simulink model "HRD05"  (R2017b)
settings: Solver=ode8  StartTime=0.0  StopTime=Inf  FixedStep=0.001  RelTol=1e-3  EnableMultiTasking=on
undefined symbols (not defined in the file or in its folder): canChannel
libraries: c280xlib x7, canmsglib x4, canlib x3, c2806xlib x3, c2000lib x1, simulink x1, simulink_extras x1
settings Model: ExtModeTrigDuration=8  Creator=koffi  LastModifiedBy=Mark
settings OptimizationCC: LifeSpan=1  MaxStackSize=512
settings DebuggingCC: SFUnexpectedBacktrackingDiag=warning  SFNoUnconditionalDefaultTransitionDiag=warning  SFExecutionAtInitializationDiag=none
settings HardwareCC: ProdBitPerChar=16  ProdBitPerInt=16  ProdBitPerPointer=32  ProdBitPerSizeT=32  ProdBitPerPtrDiffT=32  ProdLargestAtomicInteger=Integer  ProdLargestAtomicFloat=None  ProdWordSize=16  ProdLongLongMode=on  ProdHWDeviceType=Texas Instruments->C2000
settings SFSimCC: MATLABDynamicMemAlloc=off
settings RTWCC: SystemTargetFile=ert.tlc  HardwareBoard=TI Piccolo F2806x (boot from flash)  TemplateMakefile=ert_default_tmf  GenerateReport=on  Toolchain=Texas Instruments Code Composer Studio (C2000)  IncludeHyperlinkInReport=on  LaunchReport=on  GenerateTraceInfo=on  GenerateTraceReport=on  GenerateTraceReportSl=on  GenerateTraceReportSf=on  GenerateTraceReportEml=on
settings CodeAppCC: ForceParamTrailComments=on  IgnoreCustomStorageClasses=off  OperatorAnnotations=on  SimulinkDataObjDesc=on  SFDataObjDesc=on  MATLABFcnDesc=on  InsertBlockDesc=on  StateflowObjectComments=on  MATLABSourceComments=on
settings ERTTargetCC: CodeReplacementLibrary=TI C28x  MultiwordLength=2048  ExtMode=on  ExtModeTransport=1  ExtModeMexFile=ext_serial_win32_comm  ExtModeMexArgs=1 7 114796
settings ConfigComp: CovMetricSettings=dw  CovHtmlReporting=on  CovSaveCumulativeToWorkspaceVar=on  CovSaveSingleToWorkspaceVar=on  CovExternalEMLEnable=off

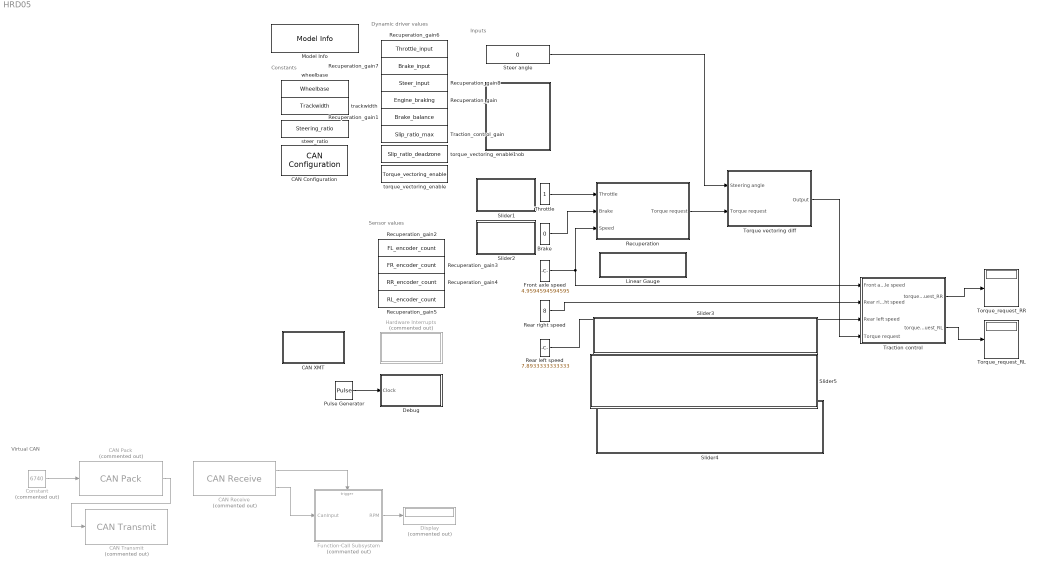
== system HRD05 ==
  note: Inputs
  note: Constants
  note: Dynamic driver values
  note: Sensor values
  note: Virtual CAN
  Brake : Constant  Value=0  OutDataTypeStr=double
  CAN Configuration : canlib/CAN Configuration  BlockHandle=5.0002  DeviceMenu=MathWorks Virtual 1 (Channel 1)  Device=MathWorks Virtual 1 (Channel 1)  ObjConstructor=canChannel('MathWorks','Virtual 1',1)  BusSpeed=500000  EnableBitParameters=off  AckMode=Normal
      settings: SourceProductName=Vehicle Network Toolbox  SourceProductBaseCode=VN
  CAN Pack : canmsglib/CAN Pack  Commented=on  CANdbFile=C:\HARD\HRD05-Control-system\config.dbc  MsgList=Engine_RPM  MsgName=Engine_RPM  MsgIDType=Standard (11-bit identifier)  MsgIdentifier=10  MsgLength=2  SignalInfo=Engine_RPM$0$15$1$2$1$0$1$0$0$32767$#  NSignals=1  StartBits=str2num('[int32(0)]')  SignalSizes=str2num('[int32(15)]')  ByteOrders=str2num('[int32(1)]')  DataTypes=str2num('[int32(2)]')  MultiplexTypes=str2num('[int32(1)]')  MultiplexValues=str2num('[double(0)]')  Factors=str2num('[double(1)]')  Offsets=str2num('[double(0)]')  Minimums=str2num('[double(0)]')  Maximums=str2num('[double(32767)]')  Remote=off  ApplyMinMax=off  BusOutput=off
      settings: SourceProductName=Simulink Real-Time  SourceProductBaseCode=XP  DataFormat=CANdb specified signals
  CAN Receive : canlib/CAN Receive  Commented=on  BlockHandle=7.0002  DeviceMenu=MathWorks Virtual 1 (Channel 1)  Device=MathWorks Virtual 1 (Channel 1)  ObjConstructor=canChannel('MathWorks','Virtual 1',1)  EnableStandardIDsFilter=off  StandardIDs=0  EnableExtendedIDsFilter=off  ExtendedIDs=0  SampleTime=0.01  MsgsPerTimestep=all  StdIDsCombo=Allow all  ExtIDsCombo=Allow all  InternalFilterUpdateStatus=on  BusOutput=off
      settings: SourceProductName=Vehicle Network Toolbox  SourceProductBaseCode=VN
  CAN Transmit : canlib/CAN Transmit  Commented=on  BlockHandle=8.0002  DeviceMenu=MathWorks Virtual 1 (Channel 1)  Device=MathWorks Virtual 1 (Channel 1)  ObjConstructor=canChannel('MathWorks','Virtual 1',1)  EnablePeriodicTransmit=off  MessagePeriod=1.000
      settings: SourceProductName=Vehicle Network Toolbox  SourceProductBaseCode=VN
  CAN XMT : Subsystem
  Constant : Constant  Commented=on  Value=6740
  Debug : Subsystem
  Display : Display  Commented=on
  Front axle speed : Constant  Value=4.9594594594595
  Function-Call Subsystem : Subsystem  Commented=on  TreatAsAtomicUnit=on
  Hardware Interrupts : Subsystem  Commented=on
  Knob : Subsystem  DialogController=hmiCreateDDGDialog  IsWebBlock=on  mask(MWDashboardBlock){webBlockId=45e470c3-09e4-44e8-ab03-ef5fc6b5f1f9, webBlockType=continuousknob, ShowInLibBrowser=on, ShowInitialText=on, HMISrcModelName=HRD05}
      mask prompts: webBlockId "WebBlock Id"; webBlockType "WebBlock Type"; HMISrcModelName "Source Model"
      mask help: SimulinkHMI:dialogs:ContinuousKnobDialogDesc
      mask Help: helpview([docroot '/mapfiles/simulink.map'], 'hmi_knob')
      mask Display:
      | if strcmp(get_param(bdroot(gcb),'BlockDiagramType'), 'library')
      |     image([(matlabroot) '/toolbox/simulink/hmi/icons/ContinuousKnob.png']);
      | end
  Linear Gauge : Subsystem  DialogController=hmiCreateDDGDialog  IsWebBlock=on  mask(MWDashboardBlock){webBlockId=bec7d255-bb7e-478d-9fdc-97f3e3b8b2d8, webBlockType=lineargauge, ShowInLibBrowser=on, ShowInitialText=on, HMISrcModelName=HRD05}
      mask prompts: webBlockId "WebBlock Id"; webBlockType "WebBlock Type"; HMISrcModelName "Source Model"
      mask help: SimulinkHMI:dialogs:LinearGaugeDialogDesc
      mask Help: helpview([docroot '/mapfiles/simulink.map'], 'hmi_linear_gauge')
      mask Display:
      | if strcmp(get_param(bdroot(gcb),'BlockDiagramType'), 'library')
      |     image([(matlabroot) '/toolbox/simulink/hmi/icons/LinearGauge.png']);
      | end
  Model Info : simulink/Model-Wide Utilities/Model Info  Frame=on  DisplayStringWithTags=|  HorizontalTextAlignment=Center  LeftAlignmentValue=0.5
      | Last edited by %<LastModifiedBy>,
      | %<LastModificationDate>
  Pulse Generator : DiscretePulseGenerator  PulseType=Time based  Period=1  PulseWidth=50
  Rear left speed : Constant  Value=7.8933333333333
  Rear right speed : Constant  Value=8
  Recuperation : Subsystem
  Recuperation_gain : DataStoreMemory  DataStoreName=Engine_braking  ReadBeforeWriteMsg=warning  WriteAfterWriteMsg=warning  WriteAfterReadMsg=warning  InitialValue=0.1  ShowAdditionalParam=off
  Recuperation_gain1 : DataStoreMemory  DataStoreName=Brake_balance  ReadBeforeWriteMsg=warning  WriteAfterWriteMsg=warning  WriteAfterReadMsg=warning  InitialValue=0.6  ShowAdditionalParam=off
  Recuperation_gain2 : DataStoreMemory  DataStoreName=FL_encoder_count  ReadBeforeWriteMsg=warning  WriteAfterWriteMsg=warning  WriteAfterReadMsg=warning  InitialValue=0.1  ShowAdditionalParam=off
  Recuperation_gain3 : DataStoreMemory  DataStoreName=FR_encoder_count  ReadBeforeWriteMsg=warning  WriteAfterWriteMsg=warning  WriteAfterReadMsg=warning  InitialValue=0.6  ShowAdditionalParam=off
  Recuperation_gain4 : DataStoreMemory  DataStoreName=RR_encoder_count  ReadBeforeWriteMsg=warning  WriteAfterWriteMsg=warning  WriteAfterReadMsg=warning  InitialValue=0.6  ShowAdditionalParam=off
  Recuperation_gain5 : DataStoreMemory  DataStoreName=RL_encoder_count  ReadBeforeWriteMsg=warning  WriteAfterWriteMsg=warning  WriteAfterReadMsg=warning  InitialValue=0.6  ShowAdditionalParam=off
  Recuperation_gain6 : DataStoreMemory  DataStoreName=Throttle_input  ReadBeforeWriteMsg=warning  WriteAfterWriteMsg=warning  WriteAfterReadMsg=warning  InitialValue=0.1  ShowAdditionalParam=off
  Recuperation_gain7 : DataStoreMemory  DataStoreName=Brake_input  ReadBeforeWriteMsg=warning  WriteAfterWriteMsg=warning  WriteAfterReadMsg=warning  InitialValue=0.1  ShowAdditionalParam=off
  Recuperation_gain8 : DataStoreMemory  DataStoreName=Steer_input  ReadBeforeWriteMsg=warning  WriteAfterWriteMsg=warning  WriteAfterReadMsg=warning  InitialValue=0.1  ShowAdditionalParam=off
  Slider1 : Subsystem  DialogController=hmiCreateDDGDialog  IsWebBlock=on  mask(MWDashboardBlock){webBlockId=6b16e8a2-996c-4c21-90ad-47c2870b8494, webBlockType=slider, ShowInLibBrowser=on, ShowInitialText=on, HMISrcModelName=HRD05}
      mask prompts: webBlockId "WebBlock Id"; webBlockType "WebBlock Type"; HMISrcModelName "Source Model"
      mask help: SimulinkHMI:dialogs:SliderDialogDesc
      mask Help: helpview([docroot '/mapfiles/simulink.map'], 'hmi_slider')
      mask Display:
      | if strcmp(get_param(bdroot(gcb),'BlockDiagramType'), 'library')
      |     image([(matlabroot) '/toolbox/simulink/hmi/icons/Slider.png']);
      | end
  Slider2 : Subsystem  DialogController=hmiCreateDDGDialog  IsWebBlock=on  mask(MWDashboardBlock){webBlockId=192e6944-36b0-45cd-ab7f-11e06ed1feff, webBlockType=slider, ShowInLibBrowser=on, ShowInitialText=on, HMISrcModelName=HRD05}
      mask prompts: webBlockId "WebBlock Id"; webBlockType "WebBlock Type"; HMISrcModelName "Source Model"
      mask help: SimulinkHMI:dialogs:SliderDialogDesc
      mask Help: helpview([docroot '/mapfiles/simulink.map'], 'hmi_slider')
      mask Display:
      | if strcmp(get_param(bdroot(gcb),'BlockDiagramType'), 'library')
      |     image([(matlabroot) '/toolbox/simulink/hmi/icons/Slider.png']);
      | end
  Slider3 : Subsystem  DialogController=hmiCreateDDGDialog  IsWebBlock=on  mask(MWDashboardBlock){webBlockId=7036d1ce-3a10-421e-b8b0-76df4fa24d80, webBlockType=slider, ShowInLibBrowser=on, ShowInitialText=on, HMISrcModelName=HRD05}
      mask prompts: webBlockId "WebBlock Id"; webBlockType "WebBlock Type"; HMISrcModelName "Source Model"
      mask help: SimulinkHMI:dialogs:SliderDialogDesc
      mask Help: helpview([docroot '/mapfiles/simulink.map'], 'hmi_slider')
      mask Display:
      | if strcmp(get_param(bdroot(gcb),'BlockDiagramType'), 'library')
      |     image([(matlabroot) '/toolbox/simulink/hmi/icons/Slider.png']);
      | end
  Slider4 : Subsystem  DialogController=hmiCreateDDGDialog  IsWebBlock=on  mask(MWDashboardBlock){webBlockId=54ff136d-0631-4094-b431-9d80d891858a, webBlockType=slider, ShowInLibBrowser=on, ShowInitialText=on, HMISrcModelName=HRD05}
      mask prompts: webBlockId "WebBlock Id"; webBlockType "WebBlock Type"; HMISrcModelName "Source Model"
      mask help: SimulinkHMI:dialogs:SliderDialogDesc
      mask Help: helpview([docroot '/mapfiles/simulink.map'], 'hmi_slider')
      mask Display:
      | if strcmp(get_param(bdroot(gcb),'BlockDiagramType'), 'library')
      |     image([(matlabroot) '/toolbox/simulink/hmi/icons/Slider.png']);
      | end
  Slider5 : Subsystem  DialogController=hmiCreateDDGDialog  IsWebBlock=on  mask(MWDashboardBlock){webBlockId=a28cbb47-1fb8-41d3-9559-6b9ff77cecec, webBlockType=slider, ShowInLibBrowser=on, ShowInitialText=on, HMISrcModelName=HRD05}
      mask prompts: webBlockId "WebBlock Id"; webBlockType "WebBlock Type"; HMISrcModelName "Source Model"
      mask help: SimulinkHMI:dialogs:SliderDialogDesc
      mask Help: helpview([docroot '/mapfiles/simulink.map'], 'hmi_slider')
      mask Display:
      | if strcmp(get_param(bdroot(gcb),'BlockDiagramType'), 'library')
      |     image([(matlabroot) '/toolbox/simulink/hmi/icons/Slider.png']);
      | end
  "Steer angle " : Constant  Value=0  OutDataTypeStr=double
  Throttle : Constant  OutDataTypeStr=double
  Torque vectoring diff : Subsystem  TreatAsAtomicUnit=on
  Torque_request_RL : Display
  Torque_request_RR : Display
  Traction control : Subsystem
  Traction_control_gain : DataStoreMemory  DataStoreName=Slip_ratio_max  ReadBeforeWriteMsg=warning  WriteAfterWriteMsg=warning  WriteAfterReadMsg=warning  InitialValue=2  ShowAdditionalParam=off
  steer_ratio : DataStoreMemory  DataStoreName=Steering_ratio  ReadBeforeWriteMsg=warning  WriteAfterWriteMsg=warning  WriteAfterReadMsg=warning  InitialValue=1.5  ShowAdditionalParam=off
  torque_vectoring_enable : DataStoreMemory  DataStoreName=Torque_vectoring_enable  ReadBeforeWriteMsg=warning  WriteAfterWriteMsg=warning  WriteAfterReadMsg=warning  InitialValue=1  ShowAdditionalParam=off
  torque_vectoring_enable1 : DataStoreMemory  DataStoreName=Slip_ratio_deadzone  ReadBeforeWriteMsg=warning  WriteAfterWriteMsg=warning  WriteAfterReadMsg=warning  InitialValue=1.12  ShowAdditionalParam=off
  trackwidth : DataStoreMemory  DataStoreName=Trackwidth  ReadBeforeWriteMsg=warning  WriteAfterWriteMsg=warning  WriteAfterReadMsg=warning  InitialValue=1.1  ShowAdditionalParam=off
  wheelbase : DataStoreMemory  DataStoreName=Wheelbase  ReadBeforeWriteMsg=warning  WriteAfterWriteMsg=warning  WriteAfterReadMsg=warning  InitialValue=1.5  ShowAdditionalParam=off
  wires:
  Brake/1 -> Recuperation/2(Brake)
  Throttle/1 -> Recuperation/1(Throttle)
  Torque vectoring diff/1("Output ") -> Traction control/4(Torque request)
  Front axle speed/1 -> Traction control/1(Front axle speed), Recuperation/3(Speed)
  Traction control/1("torque_request_RR ") -> Torque_request_RR/1
  Recuperation/1(Torque request) -> Torque vectoring diff/2(Torque request)
  Pulse Generator/1 -> Debug/1(Clock)
  CAN Receive/2 -> Function-Call Subsystem/1("CanInput ")
  Function-Call Subsystem/1(RPM) -> Display/1
  CAN Pack/1 -> CAN Transmit/1
  Constant/1 -> CAN Pack/1
  CAN Receive/1 -> Function-Call Subsystem/Trigger
  "Steer angle "/1 -> Torque vectoring diff/1(Steering angle)
  Rear left speed/1 -> Traction control/3(Rear left speed)
  Rear right speed/1 -> Traction control/2(Rear right speed)
  Traction control/2(torque_request_RL) -> Torque_request_RL/1

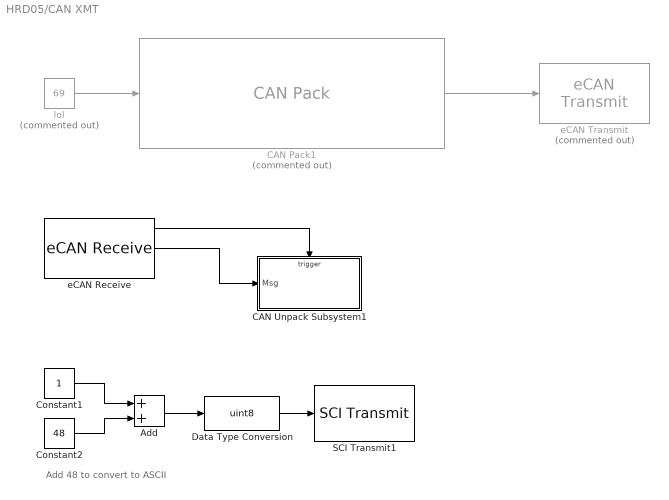
== system HRD05/CAN XMT ==
  note: Add 48 to convert to ASCII
  Add : Sum
  CAN Pack1 : canmsglib/CAN Pack  Commented=on  CANdbFile=C:\HARD\HRD05-Control-system\config.dbc  MsgList=Engine_RPM  MsgName=Engine_RPM  MsgIDType=Standard (11-bit identifier)  MsgIdentifier=10  MsgLength=2  SignalInfo=Engine_RPM$0$15$1$2$1$0$1$0$0$32767$#  NSignals=1  StartBits=str2num('[int32(0)]')  SignalSizes=str2num('[int32(15)]')  ByteOrders=str2num('[int32(1)]')  DataTypes=str2num('[int32(2)]')  MultiplexTypes=str2num('[int32(1)]')  MultiplexValues=str2num('[double(0)]')  Factors=str2num('[double(1)]')  Offsets=str2num('[double(0)]')  Minimums=str2num('[double(0)]')  Maximums=str2num('[double(32767)]')  Remote=off  ApplyMinMax=off  BusOutput=off
      settings: SourceProductName=Simulink Real-Time  DataFormat=raw data
  CAN Unpack Subsystem1 : Subsystem  TreatAsAtomicUnit=on
  Constant1 : Constant  SampleTime=-1
  Constant2 : Constant  Value=48
  Data Type Conversion : DataTypeConversion  OutDataTypeStr=uint8
  SCI Transmit1 : c280xlib/SCI Transmit  sciModule=A  dataHead='msg: '  dataTail=0  postInterrupt=off  numFifo=1
      settings: SourceProductName=Embedded Coder Support Package for Texas Instruments C2000 Processors
  eCAN Receive : c280xlib/eCAN Receive  chipFamily=C280x  useModule=eCAN_A  mailboxNo=0  messageID=18  messageType=Standard (11-bit identifier)  sampleTime=0.01  dataType=CAN_MESSAGE_TYPE  initValue=0  outputMessageLength=on  outputMessageTimeStamp=off  postInterrupt=off  interruptLine=0
      settings: SourceProductName=Embedded Coder Support Package for Texas Instruments C2000 Processors  SourceProductBaseCode=TIC2000
  eCAN Transmit : c280xlib/eCAN Transmit  Commented=on  chipFamily=C280x  useModule=eCAN_A  mailboxNo=1  messageID=bin2dec('111000111')  messageType=Standard (11-bit identifier)  enableBlockingMode=off  postInterrupt=off  interruptLine=0
      settings: SourceProductName=Embedded Coder Support Package for Texas Instruments C2000 Processors  SourceProductBaseCode=TIC2000
  "lol " : Constant  Commented=on  Value=69  OutDataTypeStr=uint16
  wires:
  "lol "/1 -> CAN Pack1/1
  CAN Pack1/1 -> eCAN Transmit/1
  eCAN Receive/2 -> CAN Unpack Subsystem1/1(Msg)
  eCAN Receive/1 -> CAN Unpack Subsystem1/Trigger
  Add/1 -> Data Type Conversion/1
  Data Type Conversion/1 -> SCI Transmit1/1
  Constant2/1 -> Add/2
  Constant1/1 -> Add/1

== system HRD05/Debug ==
  Clock : Inport
  Data Type Conversion : DataTypeConversion  OutDataTypeStr=uint8
  Digital Output : c2806xlib/Digital Output  GPIO_Number=GPIO32~GPIO39  GPIO_Bit0=off  GPIO_BIT0_Toggle=off  GPIO_Bit1=off  GPIO_BIT1_Toggle=off  GPIO_Bit2=on  GPIO_BIT2_Toggle=off  GPIO_Bit3=off  GPIO_BIT3_Toggle=off  GPIO_Bit4=off  GPIO_BIT4_Toggle=off  GPIO_Bit5=off  GPIO_BIT5_Toggle=off  GPIO_Bit6=off  GPIO_BIT6_Toggle=off  GPIO_Bit7=off  GPIO_BIT7_Toggle=off
      settings: SourceProductName=Embedded Coder Support Package for Texas Instruments C2000 Processors  SourceProductBaseCode=TIC2000
  wires:
  Clock/1 -> Data Type Conversion/1
  Data Type Conversion/1 -> Digital Output/1

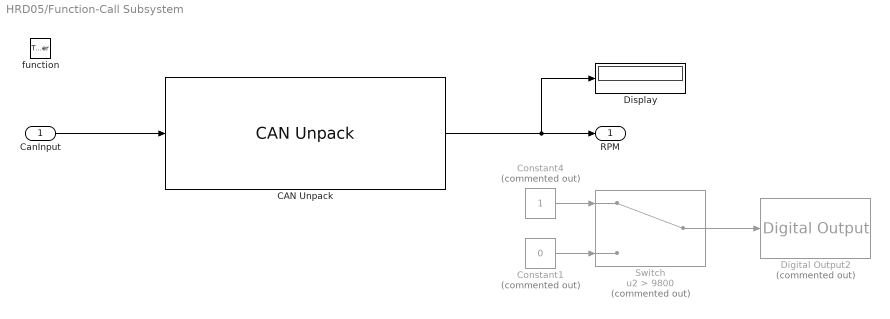
== system HRD05/Function-Call Subsystem ==
  "CanInput " : Inport
  function : TriggerPort  TriggerType=function-call  VariantControl=Variant
  CAN Unpack : canmsglib/CAN Unpack  CANdbFile=C:\HARD\HRD05-Control-system\config.dbc  MsgList=Engine_RPM  MsgName=Engine_RPM  MsgIDType=Standard (11-bit identifier)  MsgIdentifier=10  MsgLength=2  SignalInfo=Engine_RPM$0$15$1$2$1$0$1$0$0$32767$#  NSignals=1  IDPort=off  TimestampPort=off  ErrorPort=off  RemotePort=off  LengthPort=off  StatusPort=off  StartBits=str2num('[int32(0)]')  SignalSizes=str2num('[int32(15)]')  ByteOrders=str2num('[int32(1)]')  DataTypes=str2num('[int32(2)]')  MultiplexTypes=str2num('[int32(1)]')  MultiplexValues=str2num('[double(0)]')  Factors=str2num('[double(1)]')  Offsets=str2num('[double(0)]')  Minimums=str2num('[double(0)]')  Maximums=str2num('[double(32767)]')  ApplyMinMax=off
      settings: SourceProductName=Simulink Real-Time  SourceProductBaseCode=XP  DataFormat=CANdb specified signals
  Constant1 : Constant  Commented=on  Value=0  OutDataTypeStr=boolean
  Constant4 : Constant  Commented=on  OutDataTypeStr=boolean
  Digital Output2 : c2806xlib/Digital Output  Commented=on  GPIO_Number=GPIO32~GPIO39  GPIO_Bit0=off  GPIO_BIT0_Toggle=off  GPIO_Bit1=off  GPIO_BIT1_Toggle=off  GPIO_Bit2=on  GPIO_BIT2_Toggle=off  GPIO_Bit3=off  GPIO_BIT3_Toggle=off  GPIO_Bit4=off  GPIO_BIT4_Toggle=off  GPIO_Bit5=off  GPIO_BIT5_Toggle=off  GPIO_Bit6=off  GPIO_BIT6_Toggle=off  GPIO_Bit7=off  GPIO_BIT7_Toggle=off
      settings: SourceProductName=Embedded Coder Support Package for Texas Instruments C2000 Processors  SourceProductBaseCode=TIC2000
  Display : Display
  Switch : Switch  Commented=on  Criteria=u2 > Threshold  Threshold=9800
  RPM : Outport
  wires:
  "CanInput "/1 -> CAN Unpack/1
  CAN Unpack/1 -> Display/1, RPM/1
  Constant1/1 -> Switch/3
  Constant4/1 -> Switch/1
  Switch/1 -> Digital Output2/1

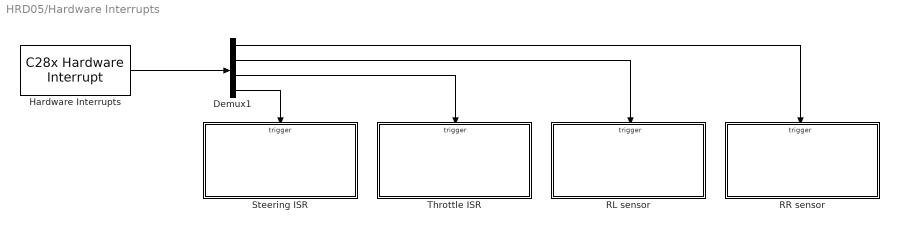
== system HRD05/Hardware Interrupts ==
  Demux1 : Demux
  Hardware Interrupts : c2000lib/Scheduling/C28x Hardware Interrupt  irqnumbers=[4 4 4 4]  pienumbers=[1 2 3 4]  irqpriorities=[25 25 2 2]  irqpreempts=[1 1 0 0]  showinput=off  dspchiptype=C280X
      settings: SourceProductName=Embedded Coder Support Package for Texas Instruments C2000 Processors  SourceProductBaseCode=TIC2000
  RL sensor : Subsystem  TreatAsAtomicUnit=on
  RR sensor : Subsystem  TreatAsAtomicUnit=on
  Steering ISR : Subsystem  TreatAsAtomicUnit=on
  Throttle ISR : Subsystem  TreatAsAtomicUnit=on
  wires:
  Hardware Interrupts/1 -> Demux1/1
  Demux1/1 -> RR sensor/Trigger
  Demux1/4 -> Steering ISR/Trigger
  Demux1/3 -> Throttle ISR/Trigger
  Demux1/2 -> RL sensor/Trigger

== system HRD05/Knob ==

== system HRD05/Linear Gauge ==

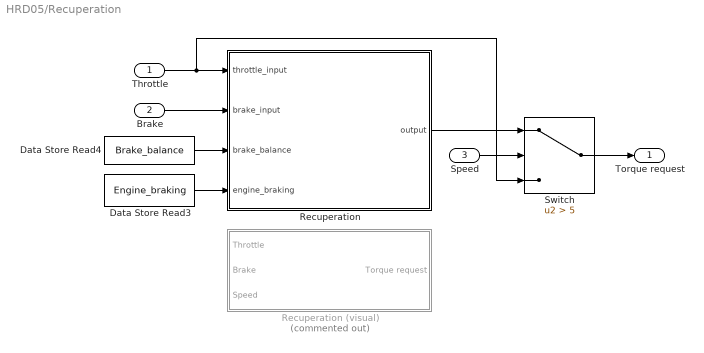
== system HRD05/Recuperation ==
  Throttle : Inport
  Brake : Inport  Port=2
  Speed : Inport  Port=3
  Data Store Read3 : DataStoreRead  DataStoreName=Engine_braking
  Data Store Read4 : DataStoreRead  DataStoreName=Brake_balance
  Recuperation : MATLAB Function  TreatAsAtomicUnit=on
  Recuperation (visual) : Subsystem  Commented=on
  Switch : Switch  Criteria=u2 > Threshold  Threshold=5
  Torque request : Outport
  wires:
  Throttle/1 -> Switch/3, Recuperation/1(throttle_input)
  Speed/1 -> Switch/2
  Recuperation/1(output) -> Switch/1
  Switch/1 -> Torque request/1
  Data Store Read4/1 -> Recuperation/3(brake_balance)
  Data Store Read3/1 -> Recuperation/4(engine_braking)
  Brake/1 -> Recuperation/2(brake_input)

== system HRD05/Slider1 ==

== system HRD05/Slider2 ==

== system HRD05/Slider3 ==

== system HRD05/Slider4 ==

== system HRD05/Slider5 ==

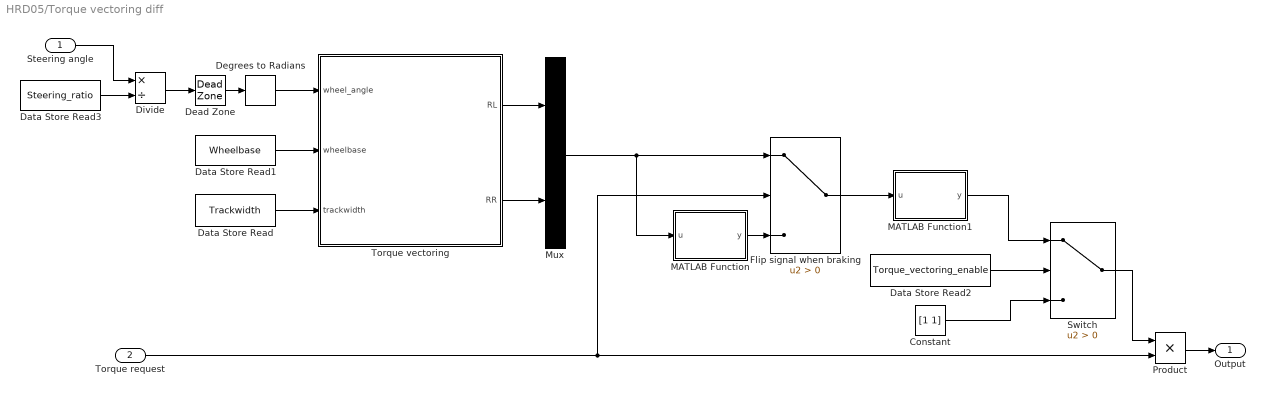
== system HRD05/Torque vectoring diff ==
  Steering angle : Inport
  Torque request : Inport  Port=2
  Constant : Constant  Value=[1 1]
  Data Store Read : DataStoreRead  DataStoreName=Trackwidth
  Data Store Read1 : DataStoreRead  DataStoreName=Wheelbase
  Data Store Read2 : DataStoreRead  DataStoreName=Torque_vectoring_enable
  Data Store Read3 : DataStoreRead  DataStoreName=Steering_ratio
  Dead Zone : DeadZone  LowerValue=-0.2  UpperValue=0.2  SaturateOnIntegerOverflow=on
  Degrees to Radians : simulink_extras/Transformations/Degrees to Radians
  Divide : Product  Inputs=*/
  Flip signal when braking : Switch  Criteria=u2 > Threshold
  MATLAB Function : MATLAB Function  TreatAsAtomicUnit=on
  MATLAB Function1 : MATLAB Function  TreatAsAtomicUnit=on
  Mux : Mux  Inputs=2
      settings: DisplayOption=signals
  Product : Product
  Switch : Switch  Criteria=u2 > Threshold
  Torque vectoring : MATLAB Function  TreatAsAtomicUnit=on
  "Output " : Outport  InitialOutput=[1 1]
  wires:
  Torque request/1 -> Flip signal when braking/2, Product/2
  MATLAB Function/1(y) -> Flip signal when braking/3
  Flip signal when braking/1 -> MATLAB Function1/1(u)
  Data Store Read2/1 -> Switch/2
  Constant/1 -> Switch/3
  Switch/1 -> Product/1
  MATLAB Function1/1(y) -> Switch/1
  Product/1 -> "Output "/1
  Data Store Read1/1 -> Torque vectoring/2(wheelbase)
  Dead Zone/1 -> Degrees to Radians/1
  Data Store Read/1 -> Torque vectoring/3(trackwidth)
  Torque vectoring/2(RR) -> Mux/2
  Torque vectoring/1(RL) -> Mux/1
  Degrees to Radians/1 -> Torque vectoring/1(wheel_angle)
  Mux/1 -> Flip signal when braking/1, MATLAB Function/1(u)
  Steering angle/1 -> Divide/1
  Data Store Read3/1 -> Divide/2
  Divide/1 -> Dead Zone/1

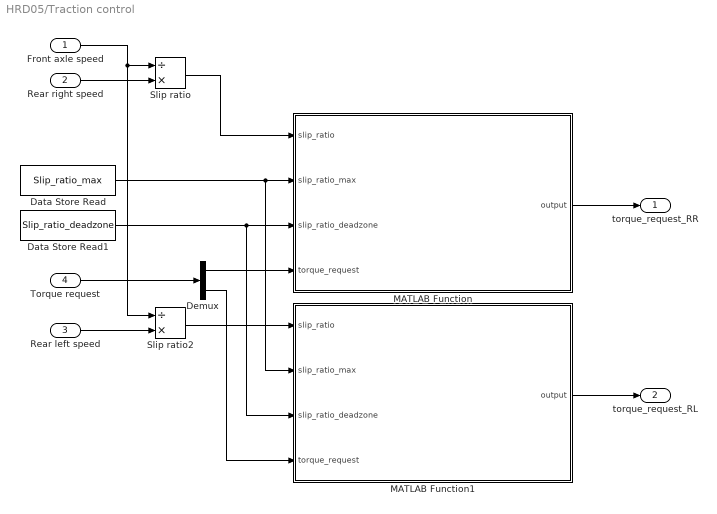
== system HRD05/Traction control ==
  Front axle speed : Inport
  Rear right speed : Inport  Port=2
  Rear left speed : Inport  Port=3
  Torque request : Inport  Port=4
  Data Store Read : DataStoreRead  DataStoreName=Slip_ratio_max
  Data Store Read1 : DataStoreRead  DataStoreName=Slip_ratio_deadzone
  Demux : Demux  Outputs=2
  MATLAB Function : MATLAB Function  TreatAsAtomicUnit=on
  MATLAB Function1 : MATLAB Function  TreatAsAtomicUnit=on
  Slip ratio : Product  Inputs=/*
  Slip ratio2 : Product  Inputs=/*
  "torque_request_RR " : Outport
  torque_request_RL : Outport  Port=2
  wires:
  MATLAB Function/1(output) -> "torque_request_RR "/1
  Torque request/1 -> Demux/1
  Front axle speed/1 -> Slip ratio2/1, Slip ratio/1
  Slip ratio/1 -> MATLAB Function/1(slip_ratio)
  Data Store Read/1 -> MATLAB Function1/2(slip_ratio_max), MATLAB Function/2(slip_ratio_max)
  Data Store Read1/1 -> MATLAB Function1/3(slip_ratio_deadzone), MATLAB Function/3(slip_ratio_deadzone)
  Demux/1 -> MATLAB Function/4(torque_request)
  Rear right speed/1 -> Slip ratio/2
  Slip ratio2/1 -> MATLAB Function1/1(slip_ratio)
  Rear left speed/1 -> Slip ratio2/2
  MATLAB Function1/1(output) -> torque_request_RL/1
  Demux/2 -> MATLAB Function1/4(torque_request)

== system HRD05/CAN XMT/CAN Unpack Subsystem1 ==
  Msg : Inport
  f : TriggerPort  TriggerType=function-call  VariantControl=Variant
  CAN Unpack : canmsglib/CAN Unpack  CANdbFile=C:\Users\josea\Desktop\C2000\CAN\Vector\RCDemo.dbc  MsgList=(none)  MsgName=Pedalbox  MsgIDType=Standard (11-bit identifier)  MsgIdentifier=18  MsgLength=2  SignalInfo=Throttle$0$8$2$1$1$0$1$0$0$255$#Brake$8$8$1$1$1$0$1$0$0$255$#  NSignals=2  IDPort=on  TimestampPort=on  ErrorPort=off  RemotePort=off  LengthPort=off  StatusPort=off  StartBits=str2num('[int32(0);int32(8)]')  SignalSizes=str2num('[int32(8);int32(8)]')  ByteOrders=str2num('[int32(2);int32(1)]')  DataTypes=str2num('[int32(1);int32(1)]')  MultiplexTypes=str2num('[int32(1);int32(1)]')  MultiplexValues=str2num('[double(0);double(0)]')  Factors=str2num('[double(1);double(1)]')  Offsets=str2num('[double(0);double(0)]')  Minimums=str2num('[double(0);double(0)]')  Maximums=str2num('[double(255);double(255)]')  ApplyMinMax=off
      settings: SourceProductName=Simulink Real-Time
  Digital Output : c2806xlib/Digital Output  Commented=on  GPIO_Number=GPIO32~GPIO39  GPIO_Bit0=off  GPIO_BIT0_Toggle=off  GPIO_Bit1=off  GPIO_BIT1_Toggle=off  GPIO_Bit2=on  GPIO_BIT2_Toggle=off  GPIO_Bit3=off  GPIO_BIT3_Toggle=off  GPIO_Bit4=off  GPIO_BIT4_Toggle=off  GPIO_Bit5=off  GPIO_BIT5_Toggle=off  GPIO_Bit6=off  GPIO_BIT6_Toggle=off  GPIO_Bit7=off  GPIO_BIT7_Toggle=off
      settings: SourceProductName=Embedded Coder Support Package for Texas Instruments C2000 Processors  SourceProductBaseCode=TIC2000
  wires:
  Msg/1 -> CAN Unpack/1
  CAN Unpack/1 -> Digital Output/1

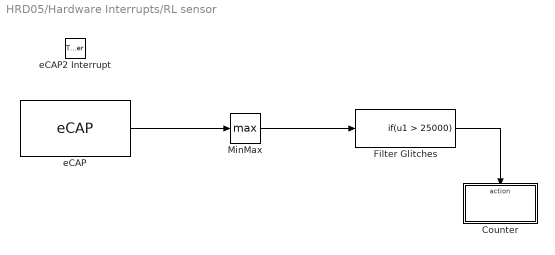
== system HRD05/Hardware Interrupts/RL sensor ==
  eCAP2 Interrupt : TriggerPort  TriggerType=function-call  VariantControl=Variant
  Counter : Subsystem  TreatAsAtomicUnit=on
  Filter Glitches : If  IfExpression=u1 > 25000  ShowElse=off
  MinMax : MinMax  Function=max
  eCAP : c280xlib/eCAP  operatingMode=eCAP  selectCAPx=eCAP2  offsetValue=0  counterSynIn=off  enableCounter=off  syncOutput=Disabled  sampleTime=-1  eventPrescaler=0  selectMode=Continuous  enableOneShot=off  stopValue=Capture Event 2  resetEv1Ts=off  ev1Polarity=Falling Edge  resetEv2Ts=on  ev2Polarity=Rising Edge  resetEv3Ts=off  ev3Polarity=Rising Edge  resetEv4Ts=on  ev4Polarity=Rising Edge  tSCntrDataType=uint32  capEvFlag=off  capFlagDataType=uint16  overFlowFlag=off  overFlowFlagDataType=uint16  periodUnit=Seconds  periodSource=Specify via dialog  waveformPeriod=0.001  dutyUnit=Percentages  dutySource=Specify via dialog  dutyCycle=50  outputPolarity=Active High  enableCEVT1Int=off  enableCEVT2Int=on  enableCEVT3Int=off  enableCEVT4Int=on  enableCTROVFInt=off  enablePRDInt=off  enableCMPInt=off
      settings: SourceProductName=Embedded Coder Support Package for Texas Instruments C2000 Processors  SourceProductBaseCode=TIC2000
  wires:
  eCAP/1 -> MinMax/1
  MinMax/1 -> Filter Glitches/1
  Filter Glitches/1 -> Counter/Action

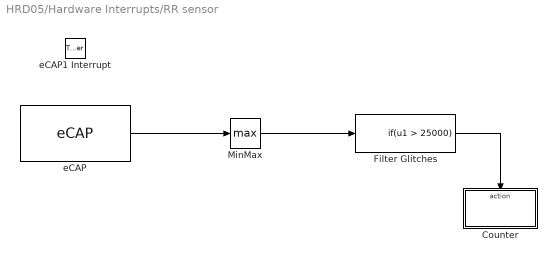
== system HRD05/Hardware Interrupts/RR sensor ==
  eCAP1 Interrupt : TriggerPort  TriggerType=function-call  VariantControl=Variant
  Counter : Subsystem  TreatAsAtomicUnit=on
  Filter Glitches : If  IfExpression=u1 > 25000  ShowElse=off
  MinMax : MinMax  Function=max
  eCAP : c280xlib/eCAP  operatingMode=eCAP  selectCAPx=eCAP1  offsetValue=0  counterSynIn=off  enableCounter=off  syncOutput=Disabled  sampleTime=-1  eventPrescaler=0  selectMode=Continuous  enableOneShot=off  stopValue=Capture Event 2  resetEv1Ts=off  ev1Polarity=Falling Edge  resetEv2Ts=on  ev2Polarity=Rising Edge  resetEv3Ts=off  ev3Polarity=Rising Edge  resetEv4Ts=on  ev4Polarity=Rising Edge  tSCntrDataType=uint32  capEvFlag=off  capFlagDataType=uint16  overFlowFlag=off  overFlowFlagDataType=uint16  periodUnit=Seconds  periodSource=Specify via dialog  waveformPeriod=0.001  dutyUnit=Percentages  dutySource=Specify via dialog  dutyCycle=50  outputPolarity=Active High  enableCEVT1Int=off  enableCEVT2Int=on  enableCEVT3Int=off  enableCEVT4Int=on  enableCTROVFInt=off  enablePRDInt=off  enableCMPInt=off
      settings: SourceProductName=Embedded Coder Support Package for Texas Instruments C2000 Processors  SourceProductBaseCode=TIC2000
  wires:
  Filter Glitches/1 -> Counter/Action
  MinMax/1 -> Filter Glitches/1
  eCAP/1 -> MinMax/1

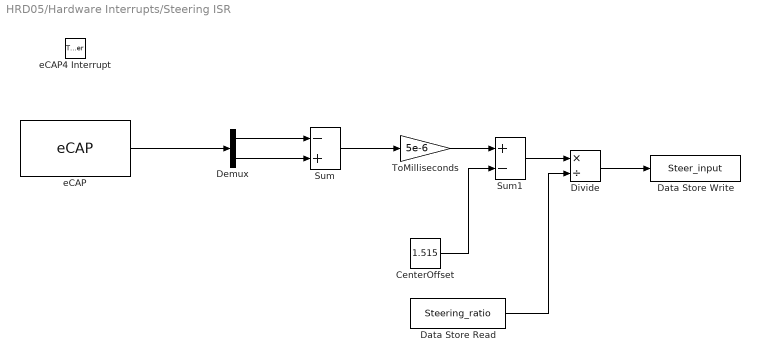
== system HRD05/Hardware Interrupts/Steering ISR ==
  eCAP4 Interrupt : TriggerPort  TriggerType=function-call  VariantControl=Variant
  CenterOffset : Constant  Value=1.515
  Data Store Read : DataStoreRead  DataStoreName=Steering_ratio
  Data Store Write : DataStoreWrite  DataStoreName=Steer_input
  Demux : Demux  Outputs=2
  Divide : Product  Inputs=*/
  Sum : Sum  Inputs=-+
  Sum1 : Sum  Inputs=+-
  ToMilliseconds : Gain  Gain=5e-6  LockScale=on
  eCAP : c280xlib/eCAP  operatingMode=eCAP  selectCAPx=eCAP1  offsetValue=0  counterSynIn=off  enableCounter=off  syncOutput=Disabled  sampleTime=-1  eventPrescaler=0  selectMode=Continuous  enableOneShot=off  stopValue=Capture Event 2  resetEv1Ts=off  ev1Polarity=Rising Edge  resetEv2Ts=off  ev2Polarity=Falling Edge  resetEv3Ts=off  ev3Polarity=Rising Edge  resetEv4Ts=on  ev4Polarity=Rising Edge  tSCntrDataType=uint32  capEvFlag=off  capFlagDataType=uint16  overFlowFlag=off  overFlowFlagDataType=uint16  periodUnit=Seconds  periodSource=Specify via dialog  waveformPeriod=0.001  dutyUnit=Percentages  dutySource=Specify via dialog  dutyCycle=50  outputPolarity=Active High  enableCEVT1Int=off  enableCEVT2Int=on  enableCEVT3Int=off  enableCEVT4Int=on  enableCTROVFInt=off  enablePRDInt=off  enableCMPInt=off
      settings: SourceProductName=Embedded Coder Support Package for Texas Instruments C2000 Processors  SourceProductBaseCode=TIC2000
  wires:
  Demux/1 -> Sum/1
  Sum/1 -> ToMilliseconds/1
  eCAP/1 -> Demux/1
  CenterOffset/1 -> Sum1/2
  ToMilliseconds/1 -> Sum1/1
  Sum1/1 -> Divide/1
  Demux/2 -> Sum/2
  Data Store Read/1 -> Divide/2
  Divide/1 -> Data Store Write/1

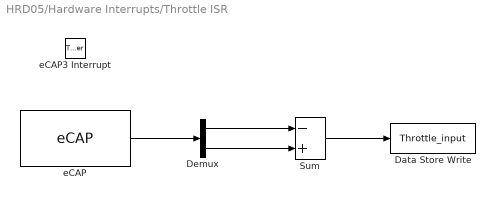
== system HRD05/Hardware Interrupts/Throttle ISR ==
  eCAP3 Interrupt : TriggerPort  TriggerType=function-call  VariantControl=Variant
  Data Store Write : DataStoreWrite  DataStoreName=Throttle_input
  Demux : Demux  Outputs=2
  Sum : Sum  Inputs=-+
  eCAP : c280xlib/eCAP  operatingMode=eCAP  selectCAPx=eCAP2  offsetValue=0  counterSynIn=off  enableCounter=off  syncOutput=Disabled  sampleTime=-1  eventPrescaler=0  selectMode=Continuous  enableOneShot=off  stopValue=Capture Event 2  resetEv1Ts=off  ev1Polarity=Rising Edge  resetEv2Ts=off  ev2Polarity=Falling Edge  resetEv3Ts=off  ev3Polarity=Rising Edge  resetEv4Ts=on  ev4Polarity=Rising Edge  tSCntrDataType=uint32  capEvFlag=off  capFlagDataType=uint16  overFlowFlag=off  overFlowFlagDataType=uint16  periodUnit=Seconds  periodSource=Specify via dialog  waveformPeriod=0.001  dutyUnit=Percentages  dutySource=Specify via dialog  dutyCycle=50  outputPolarity=Active High  enableCEVT1Int=off  enableCEVT2Int=on  enableCEVT3Int=off  enableCEVT4Int=on  enableCTROVFInt=off  enablePRDInt=off  enableCMPInt=off
      settings: SourceProductName=Embedded Coder Support Package for Texas Instruments C2000 Processors  SourceProductBaseCode=TIC2000
  wires:
  Demux/1 -> Sum/1
  eCAP/1 -> Demux/1
  Demux/2 -> Sum/2
  Sum/1 -> Data Store Write/1

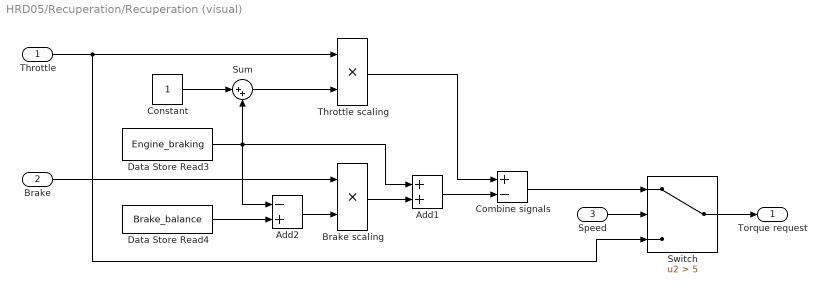
== system HRD05/Recuperation/Recuperation (visual) ==
  Throttle : Inport
  Brake : Inport  Port=2
  Speed : Inport  Port=3
  Add1 : Sum
  Add2 : Sum  Inputs=-+
  Brake scaling : Product
  Combine signals : Sum  Inputs=+-
  Constant : Constant
  Data Store Read3 : DataStoreRead  DataStoreName=Engine_braking
  Data Store Read4 : DataStoreRead  DataStoreName=Brake_balance
  Sum : Sum  Inputs=|++
  Switch : Switch  Criteria=u2 > Threshold  Threshold=5
  Throttle scaling : Product
  Torque request : Outport
  wires:
  Throttle/1 -> Switch/3, Throttle scaling/1
  Speed/1 -> Switch/2
  Brake/1 -> Brake scaling/1
  Data Store Read4/1 -> Add2/2
  Switch/1 -> Torque request/1
  Brake scaling/1 -> Add1/2
  Add1/1 -> Combine signals/2
  Data Store Read3/1 -> Add2/1, Add1/1, Sum/2
  Sum/1 -> Throttle scaling/2
  Constant/1 -> Sum/1
  Throttle scaling/1 -> Combine signals/1
  Combine signals/1 -> Switch/1
  Add2/1 -> Brake scaling/2

== system HRD05/Hardware Interrupts/RL sensor/Counter ==
  Action Port : ActionPort
  Constant : Constant  OutDataTypeStr=uint16
  Data Store Read : DataStoreRead  DataStoreName=RL_encoder_count
  Data Store Write : DataStoreWrite  DataStoreName=RL_encoder_count
  Sum1 : Sum  Inputs=|++
  wires:
  Constant/1 -> Sum1/2
  Sum1/1 -> Data Store Write/1
  Data Store Read/1 -> Sum1/1

== system HRD05/Hardware Interrupts/RR sensor/Counter ==
  Action Port : ActionPort
  Constant : Constant  OutDataTypeStr=uint16
  Data Store Read : DataStoreRead  DataStoreName=RR_encoder_count
  Data Store Write : DataStoreWrite  DataStoreName=RR_encoder_count
  Sum1 : Sum  Inputs=|++
  wires:
  Data Store Read/1 -> Sum1/1
  Sum1/1 -> Data Store Write/1
  Constant/1 -> Sum1/2

== matlab function HRD05/Recuperation/Recuperation ==
  data: throttle_input input; output output; brake_input input; brake_balance input; engine_braking input
function output = recuperation(throttle_input, brake_input, brake_balance, engine_braking)

	throttle_output = (1 + engine_braking) * throttle_input;
	brake_output = ((brake_balance - engine_braking) * brake_input) + engine_braking;

    % combine signals (-1 : 1)
    output = double(throttle_output - brake_output);

end

== matlab function HRD05/Torque vectoring diff/Torque vectoring ==
  data: wheel_angle input; wheelbase input; trackwidth input; RL output; RR output
function [RL, RR] = torque_vectoring(wheel_angle, wheelbase, trackwidth)
    
    % This block calculates all relative wheel speeds based on our Ackermann model

    % Set outputs to safe initial values
    RL = 1;
    RR = 1;
       
    % Add a small 'deadzone' to the steering input
    if abs(wheel_angle) > 0.01
    
        % Calculate x, the horizontal component of the turning circle
        x = wheelbase / tan(wheel_angle);
        
        % Calculate the radii of the rear wheels
       	RL = x + trackwidth/2;
        RR = x - trackwidth/2;
        
        % Normalize the ratios between 0 and 1
        values = [RL RR];
        ratios = abs(values / max(values));
        
        % Assign the corresponding values to each wheel
        RL = double(ratios(1));
        RR = double(ratios(2));
        
    end
    
end

== matlab function HRD05/Torque vectoring diff/MATLAB Function ==
  data: u input; y output
function y = flip(u)
y = flipud(u);

== matlab function HRD05/Torque vectoring diff/MATLAB Function1 ==
  data: u input; y output
function y = normalize(u)
y = abs(u / max(abs(u)));

== matlab function HRD05/Traction control/MATLAB Function ==
  data: slip_ratio input; slip_ratio_max input; output output; slip_ratio_deadzone input; torque_request input
function output = traction_control(slip_ratio, slip_ratio_max, slip_ratio_deadzone, torque_request)
    
    scaling = 1;
   
    if(slip_ratio > slip_ratio_deadzone)
        
        if(slip_ratio < slip_ratio_max)
            
           a = - (1 / (slip_ratio_max - slip_ratio_deadzone));
           b = 1 - (a * slip_ratio_deadzone);
           
           scaling = a * slip_ratio + b;
         
        else
            
           scaling = 0; 
           
        end
        
    end 
    
    output = torque_request * scaling;
    
end

== matlab function HRD05/Traction control/MATLAB Function1 ==
  data: slip_ratio input; slip_ratio_max input; output output; slip_ratio_deadzone input; torque_request input
function output = traction_control(slip_ratio, slip_ratio_max, slip_ratio_deadzone, torque_request)
    
    scaling = 1;
   
    if(slip_ratio > slip_ratio_deadzone)
        
        if(slip_ratio < slip_ratio_max)
            
           a = - (1 / (slip_ratio_max - slip_ratio_deadzone));
           b = 1 - (a * slip_ratio_deadzone);
           
           scaling = a * slip_ratio + b;
         
        else
            
           scaling = 0; 
           
        end
        
    end 
    
    output = torque_request * scaling;
    
end
